simulink model "Test2_Mainor"  (R2023a)
settings: Solver=FixedStepAuto  StartTime=0.0  StopTime=200  FixedStep=0.01  RelTol=1e-3
settings Model: Creator=Hp  LastModifiedBy=Hp

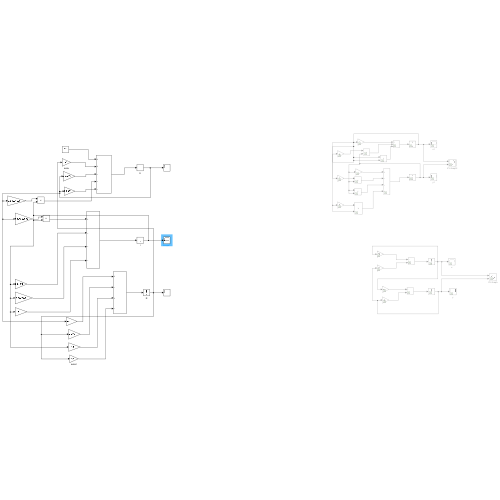
[thumbnail: Simulink's stored preview of the top-level diagram]
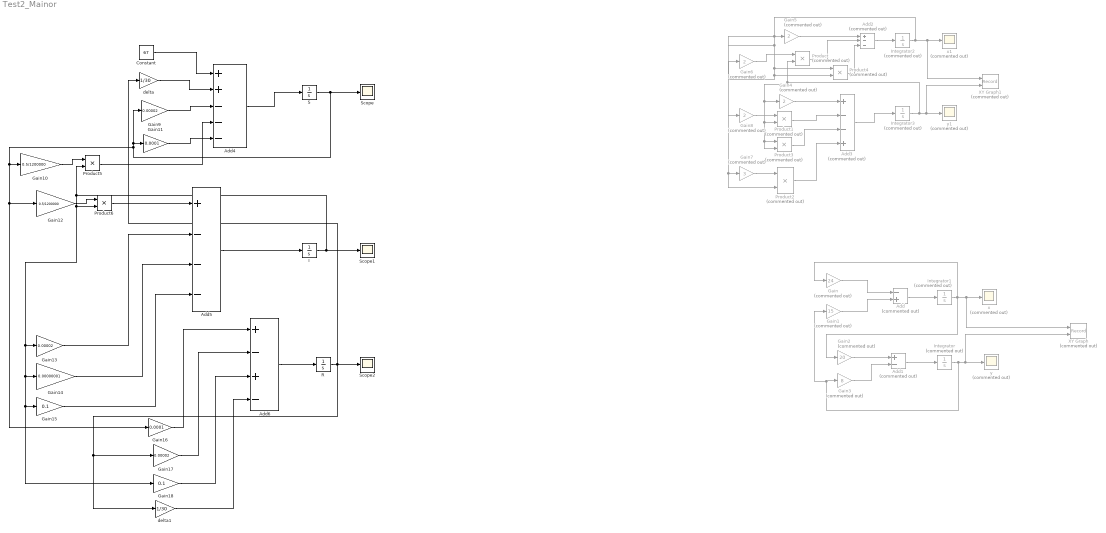
== system Test2_Mainor ==
  Add : Sum  Commented=on  Inputs=-+
  Add1 : Sum  Commented=on  Inputs=+-
  Add2 : Sum  Commented=on  Inputs=+--
  Add3 : Sum  Commented=on  Inputs=+--+
  Add4 : Sum  Inputs=++---
  Add5 : Sum  Inputs=+---
  Add6 : Sum  Inputs=+-+-
  Constant : Constant  Value=67
  Gain : Gain  Commented=on  Gain=24
  Gain1 : Gain  Commented=on  Gain=15
  Gain10 : Gain  Gain=0.5/1200000
  Gain11 : Gain  Gain=0.0001
  Gain12 : Gain  Gain=0.5/1200000
  Gain13 : Gain  Gain=0.00002
  Gain14 : Gain  Gain=0.00000001
  Gain15 : Gain  Gain=0.1
  Gain16 : Gain  Gain=0.0001
  Gain17 : Gain  Gain=0.00002
  Gain18 : Gain  Gain=0.1
  Gain2 : Gain  Commented=on  Gain=20
  Gain3 : Gain  Commented=on  Gain=8
  Gain{4..6,8} (4 alike) : Gain  Commented=on  Gain=2
  Gain7 : Gain  Commented=on  Gain=3
  Gain9 : Gain  Gain=0.00002
  I : Integrator  InitialCondition=1000
  Integrator : Integrator  Commented=on  InitialCondition=1
  Integrator1 : Integrator  Commented=on  InitialCondition=1
  Integrator2 : Integrator  Commented=on  InitialCondition=0.01
  Integrator3 : Integrator  Commented=on  InitialCondition=1.99
  Product{,1..4} (5 alike) : Product  Commented=on
  Product5 : Product
  Product6 : Product
  R : Integrator  InitialCondition=90000
  S : Integrator  InitialCondition=1109000
  Scope : Scope
  Scope1 : Scope
  Scope2 : Scope
  XY Graph : Record  Commented=on  FileSettingsInternal="{\"entries\":[{\"content\":{\"excelSettings\":{\"content\":{},\"type\":\"Streamout.ExcelSettings\"}},\"type\":\"Streamout.FileSettingStorage\",\"uuid\":\"\"}],\"packageUris\":[\"http:\\/\\/schema.mathworks.com\\/mf0\\/streamout_blocks\\/R2020a\"],\"version\":\"1.0\"}"  Layout=[1 1]  SignalsInternal="{\"entries\":[{\"content\":{\"signals\":[{\"content\":{\"blockPath\":[],\"dimensions\":[1],\"domain\":\"\",\"lineColor\":\"#a2142f\",\"plots\":[1],\"port\":1,\"sid\":[\"\"],\"signalID\":326,\"signalName\":\"Integrator1\"},\"type\":\"RecordBlkView.Signal\",\"uuid\":\"\"},{\"content\":{\"blockPath\":[],\"dimensions\":[1],\"domain\":\"\",\"lineColor\":\"#139fff\",\"plots\":[1],\"port\":2,\"sid\":[\"\"],\"signalID\":330,\"signalName\":\"Integrator\"},\"type\":\"RecordBlkView.Signal\",\"uuid\":\"\"}]},\"type\":\"RecordBlkView.InputSignals\",\"uuid\":\"\"}],\"packageUris\":[\"http:\\/\\/schema.mathworks.com\\/mf0\\/streamout_blocks\\/R2020a\"],\"version\":\"1.0\"}"  VisualizationBindings="{\"xyplotplugin\":{\"info\":[{\"series\":[{\"bindingParametersList\":[{\"parameter\":\"X-Axis\",\"signalID\":326,\"signalName\":\"Integrator1\"},{\"parameter\":\"Y-Axis\",\"signalID\":330,\"signalName\":\"Integrator\"}],\"seriesID\":11145}],\"subplotID\":1}]}}"  CompatibilityTag=XY
  XY Graph1 : Record  Commented=on  FileSettingsInternal="{\"entries\":[{\"content\":{\"excelSettings\":{\"content\":{},\"type\":\"Streamout.ExcelSettings\"}},\"type\":\"Streamout.FileSettingStorage\",\"uuid\":\"\"}],\"packageUris\":[\"http:\\/\\/schema.mathworks.com\\/mf0\\/streamout_blocks\\/R2020a\"],\"version\":\"1.0\"}"  Layout=[1 1]  SignalsInternal="{\"entries\":[{\"content\":{\"signals\":[{\"content\":{\"blockPath\":[],\"dimensions\":[1],\"domain\":\"\",\"lineColor\":\"#a2142f\",\"plots\":[1],\"port\":1,\"sid\":[\"\"],\"signalID\":334,\"signalName\":\"Integrator2\"},\"type\":\"RecordBlkView.Signal\",\"uuid\":\"\"},{\"content\":{\"blockPath\":[],\"dimensions\":[1],\"domain\":\"\",\"lineColor\":\"#139fff\",\"plots\":[1],\"port\":2,\"sid\":[\"\"],\"signalID\":338,\"signalName\":\"Integrator3\"},\"type\":\"RecordBlkView.Signal\",\"uuid\":\"\"}]},\"type\":\"RecordBlkView.InputSignals\",\"uuid\":\"\"}],\"packageUris\":[\"http:\\/\\/schema.mathworks.com\\/mf0\\/streamout_blocks\\/R2020a\"],\"version\":\"1.0\"}"  VisualizationBindings="{\"xyplotplugin\":{\"info\":[{\"series\":[{\"bindingParametersList\":[{\"parameter\":\"X-Axis\",\"signalID\":334,\"signalName\":\"Integrator2\"},{\"parameter\":\"Y-Axis\",\"signalID\":338,\"signalName\":\"Integrator3\"}],\"seriesID\":36080}],\"subplotID\":1}]}}"  CompatibilityTag=XY
  delta : Gain  Gain=1/30
  delta1 : Gain  Gain=1/30
  x : Scope  Commented=on
  x1 : Scope  Commented=on
  y : Scope  Commented=on
  y1 : Scope  Commented=on
  wires:
  Add/1 -> Integrator1/1
  Integrator1/1 -> Gain2/1, Gain/1, XY Graph/1, x/1
  Integrator/1 -> Gain1/1, Gain3/1, XY Graph/2, y/1
  Add1/1 -> Integrator/1
  Gain3/1 -> Add1/2
  Gain2/1 -> Add1/1
  Gain1/1 -> Add/2
  Gain/1 -> Add/1
  Add2/1 -> Integrator2/1
  Integrator2/1 -> XY Graph1/1, x1/1, Gain8/1, Product4/1, Product4/2, Gain6/1, Product2/2, Gain7/1, Gain5/1
  Integrator3/1 -> Product1/2, Product3/2, Product3/1, Gain4/1, Product/2, XY Graph1/2, y1/1
  Add3/1 -> Integrator3/1
  Gain5/1 -> Add2/1
  Gain6/1 -> Product/1
  Product/1 -> Add2/2
  Gain4/1 -> Add3/1
  Gain8/1 -> Product1/1
  Product1/1 -> Add3/2
  Gain7/1 -> Product2/1
  Product2/1 -> Add3/4
  Product3/1 -> Add3/3
  Product4/1 -> Add2/3
  Constant/1 -> Add4/1
  S/1 -> Gain11/1, Gain9/1, Gain16/1, Gain12/1, Gain10/1, Scope/1
  I/1 -> Scope1/1, Gain18/1, Gain15/1, Gain14/1, Gain13/1, Product6/2, Product5/2
  R/1 -> delta1/1, Gain17/1, Scope2/1, delta/1
  Add4/1 -> S/1
  Add5/1 -> I/1
  Add6/1 -> R/1
  delta/1 -> Add4/2
  Gain9/1 -> Add4/3
  Gain10/1 -> Product5/1
  Product5/1 -> Add4/4
  Gain11/1 -> Add4/5
  Product6/1 -> Add5/1
  Gain12/1 -> Product6/1
  Gain13/1 -> Add5/2
  Gain14/1 -> Add5/3
  Gain15/1 -> Add5/4
  Gain16/1 -> Add6/1
  Gain17/1 -> Add6/2
  Gain18/1 -> Add6/3
  delta1/1 -> Add6/4
